simulink subsystem "Throttle_Map_2WD_NO_FILTER_NO_REGEN"  (R2023b)
settings: Solver=VariableStepAuto  StartTime=0.0  StopTime=10.0  RelTol=1e-3
values from neighbouring files (symbols this model uses):
  k_grid_min = feval(fitresult,rpm_grid_min,voltage_grid_min)    [Motor_Tables.m]
  rpm_sweep_min = linspace(0, max(motor_constants(1,:)), RPM_resolution)    [Motor_Tables.m]
  voltage_sweep_min = linspace(min(voltages), max(voltages), V_resolution)    [Motor_Tables.m]
undefined symbols (not defined in the file or in its folder): dk_grid
settings Model: Creator=Inver  LastModifiedBy=Inver

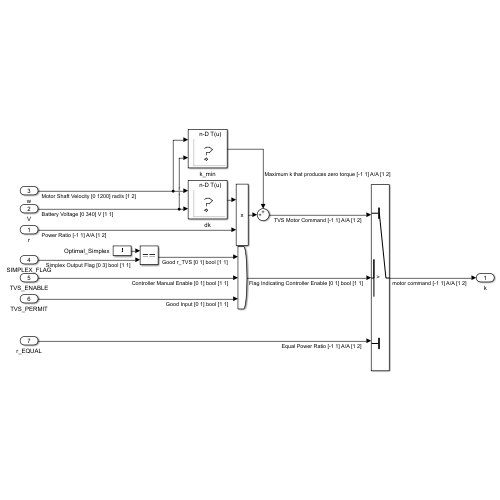
[thumbnail: Simulink's stored preview of the top-level diagram]
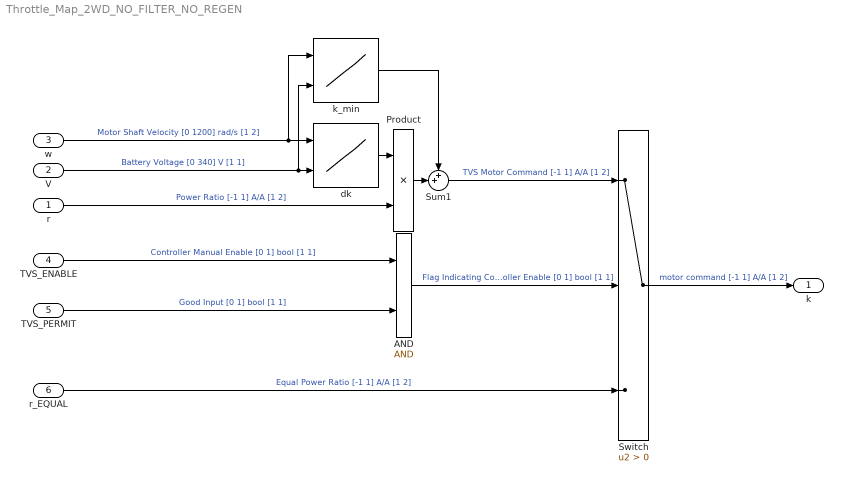
== system Throttle_Map_2WD_NO_FILTER_NO_REGEN ==
  r : Inport
  V : Inport  Port=2
  w : Inport  Port=3
  TVS_ENABLE : Inport  Port=4
  TVS_PERMIT : Inport  Port=5
  r_EQUAL : Inport  Port=6
  AND : Logic  IconShape=distinctive  AllPortsSameDT=off  OutDataTypeStr=boolean
  Product : Product
  Sum1 : Sum  Inputs=++|
  Switch : Switch  Criteria=u2 > Threshold  SaturateOnIntegerOverflow=off  InputSameDT=off
  dk : Lookup_n-D  LookupTableObject=''  BreakpointsForDimension1=rpm_sweep_min  BreakpointsForDimension2=voltage_sweep_min  BreakpointsForDimension1FirstPoint=10  BreakpointsForDimension2FirstPoint=10  BreakpointsForDimension1Spacing=12  BreakpointsForDimension2Spacing=12  IndexSearchMethod=Evenly spaced points  Table=dk_grid  ExtrapMethod=Clip  DiagnosticForOutOfRangeInput=Error  InternalRulePriority=Speed  RndMeth=Simplest
      settings: InputPortMap=u0,u1
  k_min : Lookup_n-D  LookupTableObject=''  BreakpointsForDimension1=rpm_sweep_min  BreakpointsForDimension2=voltage_sweep_min  BreakpointsForDimension1FirstPoint=10  BreakpointsForDimension2FirstPoint=10  BreakpointsForDimension1Spacing=12  BreakpointsForDimension2Spacing=12  IndexSearchMethod=Evenly spaced points  Table=k_grid_min  ExtrapMethod=Clip  DiagnosticForOutOfRangeInput=Error  InternalRulePriority=Speed  RndMeth=Simplest
      settings: InputPortMap=u0,u1
  k : Outport
  wires:
  w/1 -> dk/1, k_min/1  "Motor Shaft Velocity [0 1200] rad/s [1 2]"
  V/1 -> dk/2, k_min/2  "Battery Voltage [0 340] V [1 1]"
  r/1 -> Product/2  "Power Ratio [-1 1] A/A [1 2]"
  Sum1/1 -> Switch/1  "TVS Motor Command [-1 1] A/A [1 2]"
  k_min/1 -> Sum1/1
  dk/1 -> Product/1
  Product/1 -> Sum1/2
  Switch/1 -> k/1  "motor command [-1 1] A/A [1 2]"
  TVS_PERMIT/1 -> AND/2  "Good Input [0 1] bool [1 1]"
  TVS_ENABLE/1 -> AND/1  "Controller Manual Enable [0 1] bool [1 1]"
  AND/1 -> Switch/2  "Flag Indicating Controller Enable [0 1] bool [1 1]"
  r_EQUAL/1 -> Switch/3  "Equal Power Ratio [-1 1] A/A [1 2]"
